simulink model "cw3"  (R2023a)
settings: Solver=VariableStepAuto  StartTime=0.0  StopTime=10.0  RelTol=1e-3
libraries: spsVoltageMeasurementLib x2, spsACVoltageSourceLib x1, spsCurrentMeasurementLib x1, spsDiodeLib x1, spsSeriesRLCLoadLib x1
settings Model: Creator=student  LastModifiedBy=student

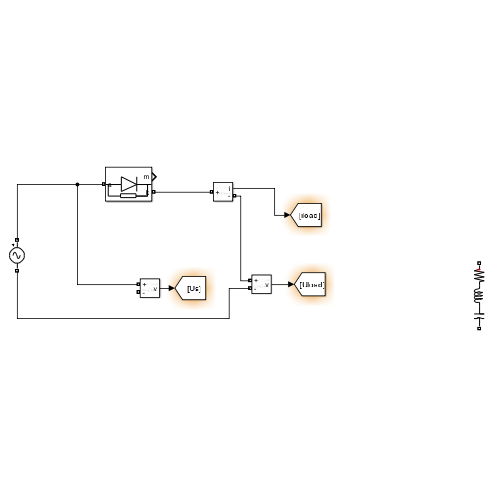
[thumbnail: Simulink's stored preview of the top-level diagram]
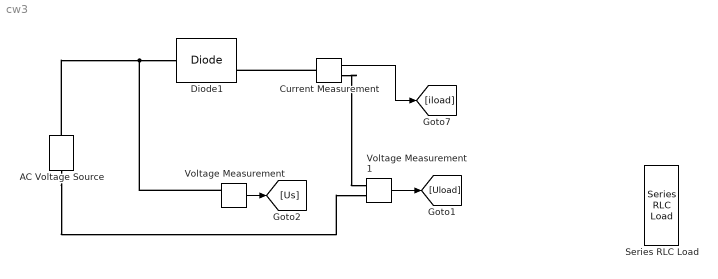
== system cw3 ==
  AC Voltage Source : spsACVoltageSourceLib/AC Voltage Source  Amplitude=100  Phase=0  Frequency=60  SampleTime=0  Measurements=None  BusType=swing  Pref=10e3  Qref=0  Qmin=-inf  Qmax=+inf
  Current Measurement : spsCurrentMeasurementLib/Current Measurement  PhasorSimulation=off  OutputType=Complex  PSBequivalent=0
  Diode1 : spsDiodeLib/Diode  Ron=0.001  Lon=0  Vf=0.8  IC=0  UseSnubber=0  Rs=500  Cs=250e-9  Measurements=on
  Series RLC Load : spsSeriesRLCLoadLib/Series RLC Load  LConnTagsString=a  RConnTagsString=__new0  NominalVoltage=1000  NominalFrequency=60  ActivePower=10e3  InductivePower=100  CapacitivePower=100  Setx0=off  InitialVoltage=0  SetiL0=off  InitialCurrent=0  Measurements=None  LoadType=constant Z
  Voltage Measurement : spsVoltageMeasurementLib/Voltage Measurement  PhasorSimulation=off  OutputType=Complex  PSBequivalent=0
  Voltage Measurement1 : spsVoltageMeasurementLib/Voltage Measurement  PhasorSimulation=off  OutputType=Complex  PSBequivalent=0
  wires:
  Voltage Measurement/1 -> [Us]
  Voltage Measurement1/1 -> [Uload]
  Current Measurement/1 -> [iload]
  connections:
  AC Voltage Source/RConn1 -- Voltage Measurement/LConn1 -- Diode1/LConn1
  Current Measurement/LConn1 -- Diode1/RConn1
  AC Voltage Source/LConn1 -- Voltage Measurement1/LConn2
  Current Measurement/RConn1 -- Voltage Measurement1/LConn1
